simulink model "Quaternions_Method_main_davide"  (R2021b)
settings: Solver=ode4  StartTime=0.0  StopTime=Time  FixedStep=1e-2  RelTol=1e-13  AbsTol=1e-8
values from neighbouring files (symbols this model uses):
  a = 8.6251e+06    (= 8625100)    [Main.m]
  c = 299792*10^3    (= 299792000)    [Main.m]
  e = 0.1195    [Main.m]
  f_mag = 18    [Main.m]
  G = 6.67259 * 1e-11    (= 6.67259e-11)    [Main.m]
  H_0 = sqrt((g_1_0)^2 + (g_1_1)^2 + (h_1_1)^2)    [Main.m]
  i = 0.3815    [Main.m]
  MB = [2000; 0.3; 1; 0.12].*1e-2    [Main.m]
  muP = G*Mt    (= 398527110340000)    [Main.m]
  omega_0 = [om_x, om_y, om_z]    [Main.m]
  p_acc = 0.5    [Main.m]
  RD = 0.1*ones(1,10)    [Main.m]
  RS_MB = 0.5    [Main.m]
  RS_SP = 0.1    [Main.m]
  SP = [2000; 0.3; 1; 0.12].*1e-2    [Main.m]
  theta0 = 0    [Main.m]
  w_E = (2*pi)/(24*3600)    (= 7.27220521664e-05)    [Main.m]
undefined symbols (not defined in the file or in its folder): A_BN_0, A_rw, A_rw_star, H, magnitude, mr, rho_d_MB, rho_s_MB, sig_b, sig_n, T, t_sample
libraries: matrix_library x18, vrlib x8, simulink x2, simulink_extras x1
(part 3 of 6)

== system Quaternions_Method_main_davide/Sensors/Magnetometer1/Magnetometer  ==
  note: Questo blocco serve a verificare ortonrmalizzazione. Per verificare la amtrice in display deve avere daigonale 1
  A_BN : Inport
  Error Matrices : Subsystem
  Matrix Multiply : Product  Inputs=4  Multiplication=Matrix(*)
  RC Low Pass FIlter : Subsystem
  orthonormalization step 1 : Subsystem
  orthonormalization step 2 : Subsystem
  orthonormalization step 3 : Subsystem
  A_BN*_filtered : Outport
  A_BN*_not_filtered : Outport  Port=2
  wires:
  A_BN/1 -> Matrix Multiply/1
  Matrix Multiply/1 -> A_BN*_not_filtered/1, RC Low Pass FIlter/1(A*)
  Error Matrices/1(A_no) -> Matrix Multiply/2
  Error Matrices/2(A_sf) -> Matrix Multiply/3
  Error Matrices/3(A_noise) -> Matrix Multiply/4
  orthonormalization step 1/1(A_BN*_filtered) -> orthonormalization step 2/1(A*(t))
  RC Low Pass FIlter/1(A*_filtered) -> orthonormalization step 1/1(A*(t))
  orthonormalization step 2/1(A_BN*_filtered) -> orthonormalization step 3/1(A*(t))
  orthonormalization step 3/1(A_BN*_filtered) -> A_BN*_filtered/1

== system Quaternions_Method_main_davide/Sensors/Magnetometer1/b_B computation ==
  A_BN* : Inport
  b_N : Inport  Port=2
  Matrix Multiply : Product  Multiplication=Matrix(*)
  Saturation : Subsystem
  b_B : Outport
  wires:
  A_BN*/1 -> Matrix Multiply/1
  b_N/1 -> Matrix Multiply/2
  Matrix Multiply/1 -> Saturation/1(b_B)
  Saturation/1(b_B saturated) -> b_B/1

== system Quaternions_Method_main_davide/Sensors/Magnetometer1/model to reality difference ==
  A_BN : Inport
  A_BN* : Inport  Port=2
  b_N : Inport  Port=3
  A_BN*1 : Inport  Port=4
  A_BN1 : InportShadow
  MatrixMultiply{,1..3} (4 alike) : Product  Multiplication=Matrix(*)
  Scope : Scope  NumInputPorts=2
  Sum : Sum  Inputs=|-|+|
  Sum1 : Sum  Inputs=|-|+|
  b_N1 : InportShadow  Port=3
  wires:
  A_BN*/1 -> MatrixMultiply/1
  b_N/1 -> MatrixMultiply1/2, MatrixMultiply/2
  A_BN/1 -> MatrixMultiply1/1
  MatrixMultiply1/1 -> Sum/1
  MatrixMultiply/1 -> Sum/2
  Sum/1 -> Scope/1
  Sum1/1 -> Scope/2
  A_BN1/1 -> MatrixMultiply3/1
  MatrixMultiply3/1 -> Sum1/1
  A_BN*1/1 -> MatrixMultiply2/1
  MatrixMultiply2/1 -> Sum1/2
  b_N1/1 -> MatrixMultiply3/2, MatrixMultiply2/2

== system Quaternions_Method_main_davide/Sun Pointing 1/Pointing error with DCM/Desired attitude ==
  S_N : Inport
  Constant : Constant  Value=0
  Constant1 : Constant  Value=0
  Constant2 : Constant
  Cross Product : matrix_library/Cross Product
      settings: SourceProductBaseCode=SL
  Mux : Mux  Inputs=3
  Reshape : Reshape  OutputDimensionality=Column vector (2-D)
  Reshape1 : Reshape  OutputDimensionality=Customize  OutputDimensions=[3,3]
  Transpose : Math  Operator=transpose  SaturateOnIntegerOverflow=on
  Vector Concatenate : Concatenate  NumInputs=3
  Desired A_B_N : Outport
  wires:
  Constant/1 -> Mux/1
  Constant1/1 -> Mux/2
  Constant2/1 -> Mux/3
  Mux/1 -> Reshape/1
  Reshape/1 -> Vector Concatenate/3, Cross Product/1
  S_N/1 -> Cross Product/2, Vector Concatenate/2
  Cross Product/1 -> Vector Concatenate/1
  Vector Concatenate/1 -> Reshape1/1
  Reshape1/1 -> Transpose/1
  Transpose/1 -> Desired A_B_N/1

== system Quaternions_Method_main_davide/Sun Pointing 1/Pointing error with DCM/Detected pointing error ==
  Desired A_B_N : Inport
  A_B_N from attitude determination : Inport  Port=2
  Add : Sum  Inputs=+|+|+
  Add1 : Sum  Inputs=+|+|+
  Demux : Demux  Outputs=9
  Demux1 : Demux  Outputs=9
  Divide : Product  Inputs=*/
  Dot Product : DotProduct  InputSameDT=on  OutDataTypeStr=Inherit: Inherit via internal rule
  Gain : Gain  Gain=180/pi
  Mux : Mux  Inputs=3
  Mux1 : Mux  Inputs=3
  Power{,1..5} (6 alike) : Math  Operator=magnitude^2  SaturateOnIntegerOverflow=on
  Product : Product
  Reshape{,1..3} (4 alike) : Reshape  OutputDimensionality=Column vector (2-D)
  Sqrt : Sqrt  SaturateOnIntegerOverflow=on
  Terminator{,1..11} (12 alike) : Terminator
  Trigonometric Function : Trigonometry  Operator=acos
  detected pointing error : Outport
  wires:
  Desired A_B_N/1 -> Reshape/1
  Reshape/1 -> Demux/1
  Demux/1 -> Terminator/1
  Demux/2 -> [A21]
  Demux/3 -> Terminator1/1
  Demux/4 -> Terminator2/1
  Demux/6 -> Terminator3/1
  Demux/7 -> Terminator4/1
  Demux/8 -> [A23]
  Demux/9 -> Terminator5/1
  Demux1/7 -> Terminator10/1
  Demux1/6 -> Terminator9/1
  Demux1/5 -> [B22]
  Demux1/3 -> Terminator7/1
  Demux1/1 -> Terminator6/1
  Demux1/8 -> [B23]
  Demux1/4 -> Terminator8/1
  Reshape1/1 -> Demux1/1
  Demux1/2 -> [B21]
  Demux1/9 -> Terminator11/1
  A_B_N from attitude determination/1 -> Reshape1/1
  [A21] -> Power/1, Mux/1
  [A22] -> Mux/2, Power1/1
  [A23] -> Mux/3, Power2/1
  Mux/1 -> Reshape2/1
  Mux1/1 -> Reshape3/1
  [B22] -> Mux1/2, Power4/1
  [B21] -> Power5/1, Mux1/1
  [B23] -> Mux1/3, Power3/1
  Reshape2/1 -> Dot Product/1
  Reshape3/1 -> Dot Product/2
  Dot Product/1 -> Divide/1
  Power1/1 -> Add/2
  Power2/1 -> Add/1
  Power/1 -> Add/3
  Add/1 -> Sqrt/1
  Sqrt/1 -> Product/1
  Power4/1 -> Add1/2
  Power5/1 -> Add1/1
  Power3/1 -> Add1/3
  Add1/1 -> Product/2
  Product/1 -> Divide/2
  Divide/1 -> Trigonometric Function/1
  Trigonometric Function/1 -> Gain/1
  Gain/1 -> detected pointing error/1
  Demux/5 -> [A22]

== system Quaternions_Method_main_davide/Sun Pointing 1/Pointing error with DCM/Real pointing error ==
  " A_B_N from Euler" : Inport
  Desired A_B_N : Inport  Port=2
  Add : Sum  Inputs=+|+|+
  Add1 : Sum  Inputs=+|+|+
  Demux : Demux  Outputs=9
  Demux1 : Demux  Outputs=9
  Divide : Product  Inputs=/*
  Dot Product : DotProduct  InputSameDT=on  OutDataTypeStr=Inherit: Inherit via internal rule
  Mux : Mux  Inputs=3
  Mux1 : Mux  Inputs=3
  Power{,1..5} (6 alike) : Math  Operator=magnitude^2  SaturateOnIntegerOverflow=on
  Product : Product
  Reshape{,1..3} (4 alike) : Reshape  OutputDimensionality=Column vector (2-D)
  Sqrt : Sqrt  SaturateOnIntegerOverflow=on
  Terminator{,1..11} (12 alike) : Terminator
  Trigonometric Function : Trigonometry  Operator=acos
  real pointing error : Outport
  wires:
  Divide/1 -> Trigonometric Function/1
  Product/1 -> Divide/1
  Add1/1 -> Product/2
  Power3/1 -> Add1/3
  Power5/1 -> Add1/1
  Power4/1 -> Add1/2
  Sqrt/1 -> Product/1
  Add/1 -> Sqrt/1
  Power/1 -> Add/3
  Power2/1 -> Add/1
  Power1/1 -> Add/2
  Dot Product/1 -> Divide/2
  Reshape3/1 -> Dot Product/2
  Reshape2/1 -> Dot Product/1
  [B23] -> Power3/1, Mux1/3
  [B21] -> Mux1/1, Power5/1
  [B22] -> Power4/1, Mux1/2
  Mux1/1 -> Reshape3/1
  Mux/1 -> Reshape2/1
  [A23] -> Power2/1, Mux/3
  [A22] -> Power1/1, Mux/2
  [A21] -> Mux/1, Power/1
  Desired A_B_N/1 -> Reshape1/1
  Demux1/9 -> Terminator11/1
  Demux1/2 -> [B21]
  Reshape1/1 -> Demux1/1
  Demux1/4 -> Terminator8/1
  Demux1/8 -> [B23]
  Demux1/1 -> Terminator6/1
  Demux1/3 -> Terminator7/1
  Demux1/5 -> [B22]
  Demux1/6 -> Terminator9/1
  Demux1/7 -> Terminator10/1
  Demux/9 -> Terminator5/1
  Demux/8 -> [A23]
  Demux/7 -> Terminator4/1
  Demux/6 -> Terminator3/1
  Demux/5 -> [A22]
  Demux/4 -> Terminator2/1
  Demux/3 -> Terminator1/1
  Demux/2 -> [A21]
  Demux/1 -> Terminator/1
  Reshape/1 -> Demux/1
  " A_B_N from Euler"/1 -> Reshape/1
  Trigonometric Function/1 -> real pointing error/1

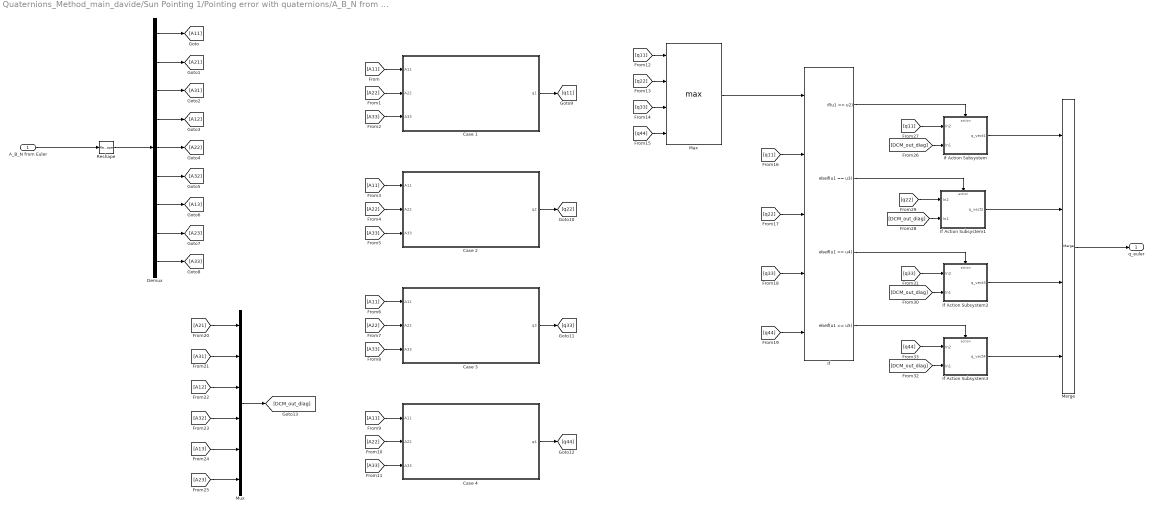
== system Quaternions_Method_main_davide/Sun Pointing 1/Pointing error with quaternions/A_B_N from Euler to quaternion ==
  A_B_N from Euler : Inport
  Case 1 : Subsystem
  Case 2 : Subsystem
  Case 3 : Subsystem
  Case 4 : Subsystem
  Demux : Demux  Outputs=9
  If : If  NumInputs=5  IfExpression=u1 == u2  ElseIfExpressions=u1 == u3, u1 == u4, u1 == u5  ShowElse=off
  If Action Subsystem : Subsystem  TreatAsAtomicUnit=on
  If Action Subsystem1 : Subsystem  TreatAsAtomicUnit=on
  If Action Subsystem2 : Subsystem  TreatAsAtomicUnit=on
  If Action Subsystem3 : Subsystem  TreatAsAtomicUnit=on
  Max : MinMax  Function=max  Inputs=4
  Merge : Merge  Inputs=4
  Mux : Mux  Inputs=6
  Reshape : Reshape  OutputDimensionality=Column vector (2-D)
  q_euler : Outport
  wires:
  A_B_N from Euler/1 -> Reshape/1
  Reshape/1 -> Demux/1
  Demux/1 -> [A11]
  Demux/2 -> [A21]
  Demux/3 -> [A31]
  Demux/4 -> [A12]
  Demux/5 -> [A22]
  Demux/6 -> [A32]
  Demux/7 -> [A13]
  Demux/8 -> [A23]
  Demux/9 -> [A33]
  [A22] -> Case 1/2(A22)
  [A33] -> Case 1/3(A33)
  [A11] -> Case 1/1(A11)
  [A11] -> Case 2/1(A11)
  [A33] -> Case 2/3(A33)
  [A22] -> Case 2/2(A22)
  [A22] -> Case 3/2(A22)
  [A33] -> Case 3/3(A33)
  [A11] -> Case 3/1(A11)
  [A11] -> Case 4/1(A11)
  [A33] -> Case 4/3(A33)
  [A22] -> Case 4/2(A22)
  Case 1/1(q1) -> [q11]
  Case 2/1(q2) -> [q22]
  Case 3/1(q3) -> [q33]
  Case 4/1(q4) -> [q44]
  [q11] -> Max/1
  [q33] -> Max/3
  [q22] -> Max/2
  [q44] -> Max/4
  Max/1 -> If/1
  [q11] -> If/2
  [q22] -> If/3
  [q33] -> If/4
  [q44] -> If/5
  If/1 -> If Action Subsystem/Action
  If/2 -> If Action Subsystem1/Action
  If/3 -> If Action Subsystem2/Action
  If/4 -> If Action Subsystem3/Action
  If Action Subsystem3/1(q_vect4) -> Merge/4
  If Action Subsystem2/1(q_vect3) -> Merge/3
  If Action Subsystem1/1(q_vect2) -> Merge/2
  If Action Subsystem/1(q_vect1) -> Merge/1
  Merge/1 -> q_euler/1
  [A23] -> Mux/6
  [A13] -> Mux/5
  [A32] -> Mux/4
  [A12] -> Mux/3
  [A31] -> Mux/2
  [A21] -> Mux/1
  Mux/1 -> [DCM_out_diag]
  [DCM_out_diag] -> If Action Subsystem/2(In1)
  [q11] -> If Action Subsystem/1(In2)
  [q22] -> If Action Subsystem1/1(In2)
  [DCM_out_diag] -> If Action Subsystem1/2(In1)
  [DCM_out_diag] -> If Action Subsystem2/2(In1)
  [q33] -> If Action Subsystem2/1(In2)
  [q44] -> If Action Subsystem3/1(In2)
  [DCM_out_diag] -> If Action Subsystem3/2(In1)

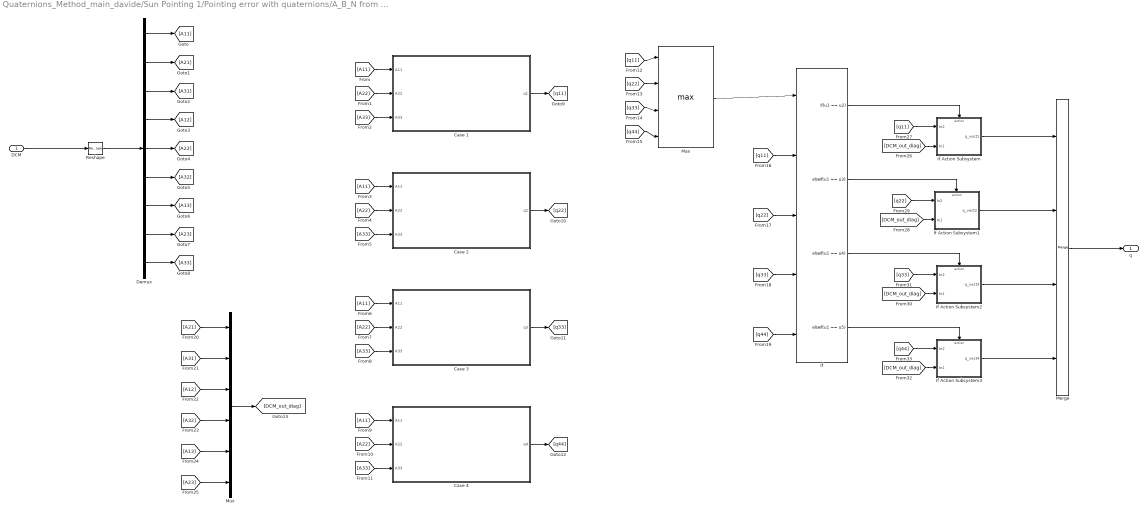
== system Quaternions_Method_main_davide/Sun Pointing 1/Pointing error with quaternions/A_B_N from attitude det to quaternion2 ==
  DCM : Inport
  Case 1 : Subsystem
  Case 2 : Subsystem
  Case 3 : Subsystem
  Case 4 : Subsystem
  Demux : Demux  Outputs=9
  If : If  NumInputs=5  IfExpression=u1 == u2  ElseIfExpressions=u1 == u3, u1 == u4, u1 == u5  ShowElse=off
  If Action Subsystem : Subsystem  TreatAsAtomicUnit=on
  If Action Subsystem1 : Subsystem  TreatAsAtomicUnit=on
  If Action Subsystem2 : Subsystem  TreatAsAtomicUnit=on
  If Action Subsystem3 : Subsystem  TreatAsAtomicUnit=on
  Max : MinMax  Function=max  Inputs=4
  Merge : Merge  Inputs=4
  Mux : Mux  Inputs=6
  Reshape : Reshape  OutputDimensionality=Column vector (2-D)
  q : Outport
  wires:
  [DCM_out_diag] -> If Action Subsystem3/2(In1)
  [q44] -> If Action Subsystem3/1(In2)
  [q33] -> If Action Subsystem2/1(In2)
  [DCM_out_diag] -> If Action Subsystem2/2(In1)
  [DCM_out_diag] -> If Action Subsystem1/2(In1)
  [q22] -> If Action Subsystem1/1(In2)
  [q11] -> If Action Subsystem/1(In2)
  [DCM_out_diag] -> If Action Subsystem/2(In1)
  Mux/1 -> [DCM_out_diag]
  [A21] -> Mux/1
  [A31] -> Mux/2
  [A12] -> Mux/3
  [A32] -> Mux/4
  [A13] -> Mux/5
  [A23] -> Mux/6
  Merge/1 -> q/1
  If Action Subsystem/1(q_vect1) -> Merge/1
  If Action Subsystem1/1(q_vect2) -> Merge/2
  If Action Subsystem2/1(q_vect3) -> Merge/3
  If Action Subsystem3/1(q_vect4) -> Merge/4
  If/4 -> If Action Subsystem3/Action
  If/3 -> If Action Subsystem2/Action
  If/2 -> If Action Subsystem1/Action
  If/1 -> If Action Subsystem/Action
  [q44] -> If/5
  [q33] -> If/4
  [q22] -> If/3
  [q11] -> If/2
  Max/1 -> If/1
  [q44] -> Max/4
  [q22] -> Max/2
  [q33] -> Max/3
  [q11] -> Max/1
  Case 4/1(q4) -> [q44]
  Case 3/1(q3) -> [q33]
  Case 2/1(q2) -> [q22]
  Case 1/1(q1) -> [q11]
  [A22] -> Case 4/2(A22)
  [A33] -> Case 4/3(A33)
  [A11] -> Case 4/1(A11)
  [A11] -> Case 3/1(A11)
  [A33] -> Case 3/3(A33)
  [A22] -> Case 3/2(A22)
  [A22] -> Case 2/2(A22)
  [A33] -> Case 2/3(A33)
  [A11] -> Case 2/1(A11)
  [A11] -> Case 1/1(A11)
  [A33] -> Case 1/3(A33)
  [A22] -> Case 1/2(A22)
  Demux/9 -> [A33]
  Demux/8 -> [A23]
  Demux/7 -> [A13]
  Demux/6 -> [A32]
  Demux/5 -> [A22]
  Demux/4 -> [A12]
  Demux/3 -> [A31]
  Demux/2 -> [A21]
  Demux/1 -> [A11]
  Reshape/1 -> Demux/1
  DCM/1 -> Reshape/1

== system Quaternions_Method_main_davide/Sun Pointing 1/Pointing error with quaternions/Desired attitude ==
  S_N : Inport
  Constant : Constant  Value=0
  Constant1 : Constant  Value=0
  Constant2 : Constant
  Cross Product : matrix_library/Cross Product
      settings: SourceProductBaseCode=SL
  Mux : Mux  Inputs=3
  Reshape : Reshape  OutputDimensionality=Column vector (2-D)
  Reshape1 : Reshape  OutputDimensionality=Customize  OutputDimensions=[3,3]
  Transpose : Math  Operator=transpose  SaturateOnIntegerOverflow=on
  Vector Concatenate : Concatenate  NumInputs=3
  Desired A_B_N : Outport
  wires:
  Constant/1 -> Mux/1
  Constant1/1 -> Mux/2
  Constant2/1 -> Mux/3
  Mux/1 -> Reshape/1
  Reshape/1 -> Cross Product/2, Vector Concatenate/3
  S_N/1 -> Vector Concatenate/2, Cross Product/1
  Cross Product/1 -> Vector Concatenate/1
  Vector Concatenate/1 -> Reshape1/1
  Reshape1/1 -> Transpose/1
  Transpose/1 -> Desired A_B_N/1

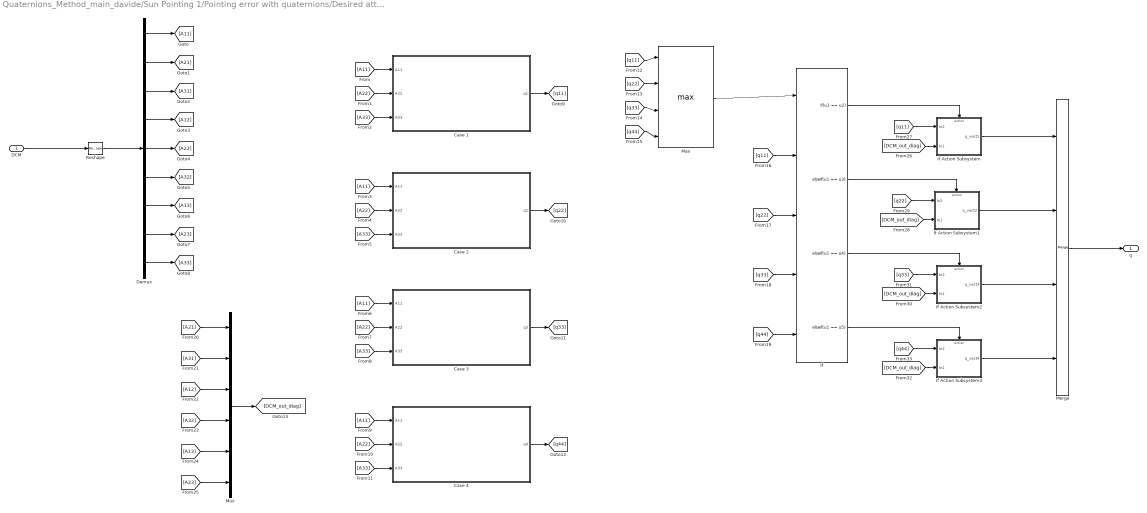
== system Quaternions_Method_main_davide/Sun Pointing 1/Pointing error with quaternions/Desired attitude to quaternion1 ==
  DCM : Inport
  Case 1 : Subsystem
  Case 2 : Subsystem
  Case 3 : Subsystem
  Case 4 : Subsystem
  Demux : Demux  Outputs=9
  If : If  NumInputs=5  IfExpression=u1 == u2  ElseIfExpressions=u1 == u3, u1 == u4, u1 == u5  ShowElse=off
  If Action Subsystem : Subsystem  TreatAsAtomicUnit=on
  If Action Subsystem1 : Subsystem  TreatAsAtomicUnit=on
  If Action Subsystem2 : Subsystem  TreatAsAtomicUnit=on
  If Action Subsystem3 : Subsystem  TreatAsAtomicUnit=on
  Max : MinMax  Function=max  Inputs=4
  Merge : Merge  Inputs=4
  Mux : Mux  Inputs=6
  Reshape : Reshape  OutputDimensionality=Column vector (2-D)
  q : Outport
  wires:
  DCM/1 -> Reshape/1
  Reshape/1 -> Demux/1
  Demux/1 -> [A11]
  Demux/2 -> [A21]
  Demux/3 -> [A31]
  Demux/4 -> [A12]
  Demux/5 -> [A22]
  Demux/6 -> [A32]
  Demux/7 -> [A13]
  Demux/8 -> [A23]
  Demux/9 -> [A33]
  [A22] -> Case 1/2(A22)
  [A33] -> Case 1/3(A33)
  [A11] -> Case 1/1(A11)
  [A11] -> Case 2/1(A11)
  [A33] -> Case 2/3(A33)
  [A22] -> Case 2/2(A22)
  [A22] -> Case 3/2(A22)
  [A33] -> Case 3/3(A33)
  [A11] -> Case 3/1(A11)
  [A11] -> Case 4/1(A11)
  [A33] -> Case 4/3(A33)
  [A22] -> Case 4/2(A22)
  Case 1/1(q1) -> [q11]
  Case 2/1(q2) -> [q22]
  Case 3/1(q3) -> [q33]
  Case 4/1(q4) -> [q44]
  [q11] -> Max/1
  [q33] -> Max/3
  [q22] -> Max/2
  [q44] -> Max/4
  Max/1 -> If/1
  [q11] -> If/2
  [q22] -> If/3
  [q33] -> If/4
  [q44] -> If/5
  If/1 -> If Action Subsystem/Action
  If/2 -> If Action Subsystem1/Action
  If/3 -> If Action Subsystem2/Action
  If/4 -> If Action Subsystem3/Action
  If Action Subsystem3/1(q_vect4) -> Merge/4
  If Action Subsystem2/1(q_vect3) -> Merge/3
  If Action Subsystem1/1(q_vect2) -> Merge/2
  If Action Subsystem/1(q_vect1) -> Merge/1
  Merge/1 -> q/1
  [A23] -> Mux/6
  [A13] -> Mux/5
  [A32] -> Mux/4
  [A12] -> Mux/3
  [A31] -> Mux/2
  [A21] -> Mux/1
  Mux/1 -> [DCM_out_diag]
  [DCM_out_diag] -> If Action Subsystem/2(In1)
  [q11] -> If Action Subsystem/1(In2)
  [q22] -> If Action Subsystem1/1(In2)
  [DCM_out_diag] -> If Action Subsystem1/2(In1)
  [DCM_out_diag] -> If Action Subsystem2/2(In1)
  [q33] -> If Action Subsystem2/1(In2)
  [q44] -> If Action Subsystem3/1(In2)
  [DCM_out_diag] -> If Action Subsystem3/2(In1)

== system Quaternions_Method_main_davide/Enviroment/Magnetic torque /Magnetic field in body frame/Direction of M field ==
  Clock : Clock
  Constant : Constant  Value=eps
  Constant1 : Constant  Value=w_E
  Mux : Mux  Inputs=3
  Product : Product
  Product1 : Product
  Product2 : Product
  Reshape : Reshape  OutputDimensionality=Column vector (2-D)
  Trigonometric Function : Trigonometry
  Trigonometric Function1 : Trigonometry  Operator=cos
  Trigonometric Function2 : Trigonometry  Operator=cos
  Trigonometric Function3 : Trigonometry
  m_vect : Outport
  wires:
  Constant1/1 -> Product/1
  Clock/1 -> Product/2
  Constant/1 -> Trigonometric Function2/1, Trigonometric Function/1
  Product/1 -> Trigonometric Function3/1, Trigonometric Function1/1
  Trigonometric Function/1 -> Product2/1, Product1/1
  Trigonometric Function1/1 -> Product1/2
  Trigonometric Function3/1 -> Product2/2
  Product1/1 -> Mux/1
  Product2/1 -> Mux/2
  Trigonometric Function2/1 -> Mux/3
  Mux/1 -> Reshape/1
  Reshape/1 -> m_vect/1

== system Quaternions_Method_main_davide/Enviroment/Solar Radiation Perturbation/Force/MB Forces ==
  P : Inport
  S_B : Inport  Port=2
  RD_MB : Inport  Port=3
  N_MB : Inport  Port=4
  M_B : Inport  Port=5
  Add : Sum
  Constant : Constant
  Constant10 : Constant  Value=[1,1,1,1,1,1]
  Constant14 : Constant  Value=[1 1 1]
  Constant4 : Constant  Value=RS_MB
  Constant8 : Constant  Value=[1 1 1]
  Constant9 : Constant  Value=[1 1 1]
  Dot Product N*MB : Subsystem
  Gain : Gain  Gain=-1
  Gain1 : Gain  Gain=2
  Gain2 : Gain  Gain=2/3
  Matrix Multiply{,1,4,6} (4 alike) : Product  Multiplication=Matrix(*)
  Product : Product  Inputs=4
  Product1 : Product
  Product2 : Product
  Product3 : Product
  Reshape : Reshape  OutputDimensionality=Column vector (2-D)
  Reshape1 : Reshape  OutputDimensionality=Row vector (2-D)
  Reshape14 : Reshape  OutputDimensionality=Column vector (2-D)
  Reshape2 : Reshape  OutputDimensionality=Row vector (2-D)
  Reshape7 : Reshape  OutputDimensionality=Row vector (2-D)
  Sum : Sum  Inputs=+-
  Sum1 : Sum
  Vector Concatenate6 : Concatenate  NumInputs=6
  creation of the areas of the S/C : Subsystem
  F_MB : Outport
  A_MB : Outport  Port=2
  prodsca_MB : Outport  Port=3
  wires:
  Constant4/1 -> Sum/2, Gain1/1
  Matrix Multiply6/1 -> Add/1
  Vector Concatenate6/1 -> Reshape14/1
  Constant9/1 -> Reshape1/1
  Reshape1/1 -> Matrix Multiply1/2
  Constant/1 -> Sum/1
  Reshape2/1 -> Matrix Multiply/2
  Gain/1 -> Product/1
  [S_B] -> Product1/1
  Sum/1 -> Product1/2
  creation of the areas of the S/C/1(a*b_1) -> Vector Concatenate6/1
  Add/1 -> Product/4
  Constant8/1 -> Reshape2/1
  Gain2/1 -> Sum1/2
  [dot_N_MB_SB] -> prodsca_MB/1
  [RD_MB] -> Gain2/1
  creation of the areas of the S/C/2(a*b_2) -> Vector Concatenate6/2
  [P] -> Gain/1
  Product2/1 -> Sum1/1
  Matrix Multiply/1 -> Product3/2
  [dot_N_MB_SB] -> Matrix Multiply1/1
  Matrix Multiply4/1 -> Product/2
  Reshape14/1 -> A_MB/1, Matrix Multiply4/1
  Matrix Multiply1/1 -> Product/3
  Gain1/1 -> Product2/2
  Sum1/1 -> Matrix Multiply/1
  creation of the areas of the S/C/4(a*h_2) -> Vector Concatenate6/4
  [dot_N_MB_SB] -> Product2/1
  creation of the areas of the S/C/5(b*h_1) -> Vector Concatenate6/5
  creation of the areas of the S/C/6(b*h_2) -> Vector Concatenate6/6
  Product1/1 -> Matrix Multiply6/2
  creation of the areas of the S/C/3(a*h_1) -> Vector Concatenate6/3
  [MB] -> creation of the areas of the S/C/1(MB)
  Constant14/1 -> Reshape7/1
  Product/1 -> F_MB/1
  Reshape7/1 -> Matrix Multiply4/2
  Product3/1 -> Add/2
  Constant10/1 -> Reshape/1
  Reshape/1 -> Matrix Multiply6/1
  [N_MB] -> Product3/1
  Dot Product N*MB/1(Out1) -> [dot_N_MB_SB]
  S_B/1 -> [S_B]
  RD_MB/1 -> [RD_MB]
  P/1 -> [P]
  N_MB/1 -> [N_MB]
  M_B/1 -> [MB]
  [S_B] -> Dot Product N*MB/1(S_B)
  [N_MB] -> Dot Product N*MB/2(N_MB)

== system Quaternions_Method_main_davide/Enviroment/Solar Radiation Perturbation/Force/SP Forces ==
  P : Inport
  S_B : Inport  Port=2
  RD_SP : Inport  Port=3
  N_SP : Inport  Port=4
  SP : Inport  Port=5
  Add1 : Sum
  Constant1 : Constant
  Constant12 : Constant  Value=[1 1 1]
  Constant13 : Constant  Value=[1 1 1]
  Constant14 : Constant  Value=[1 1 1]
  Constant15 : Constant  Value=[1,1,1,1]
  Constant5 : Constant  Value=RS_SP
  Dot Product N*SP : Subsystem
  Gain4 : Gain  Gain=-1
  Gain5 : Gain  Gain=2
  Gain6 : Gain  Gain=2/3
  Matrix Multiply{2..4,8} (4 alike) : Product  Multiplication=Matrix(*)
  Product4 : Product  Inputs=4
  Product5 : Product
  Product6 : Product
  Product7 : Product
  Reshape14 : Reshape  OutputDimensionality=Column vector (2-D)
  Reshape3 : Reshape  OutputDimensionality=Row vector (2-D)
  Reshape6 : Reshape  OutputDimensionality=Row vector (2-D)
  Reshape7 : Reshape  OutputDimensionality=Row vector (2-D)
  Reshape9 : Reshape  OutputDimensionality=Column vector (2-D)
  Sum3 : Sum  Inputs=+-
  Sum4 : Sum
  Vector Concatenate6 : Concatenate  NumInputs=4
  creation of the areas of the S/C : Subsystem
  F_SP : Outport
  prodscal_SP1 : Outport  Port=2
  wires:
  Sum3/1 -> Product5/2
  Reshape3/1 -> Matrix Multiply2/2
  Constant13/1 -> Reshape6/1
  Gain4/1 -> Product4/1
  Product6/1 -> Sum4/1
  Constant12/1 -> Reshape3/1
  [S_B] -> Product5/1
  [P] -> Gain4/1
  Gain6/1 -> Sum4/2
  [RD_SP] -> Gain6/1
  [N_SP] -> Product7/1
  Constant1/1 -> Sum3/1
  Constant15/1 -> Reshape9/1
  Sum4/1 -> Matrix Multiply3/1
  Product4/1 -> F_SP/1
  Constant5/1 -> Gain5/1, Sum3/2
  [dot_N_SP_SB] -> Matrix Multiply2/1
  Reshape6/1 -> Matrix Multiply3/2
  Product5/1 -> Matrix Multiply8/2
  Matrix Multiply3/1 -> Product7/2
  Gain5/1 -> Product6/2
  Matrix Multiply2/1 -> Product4/3
  Reshape9/1 -> Matrix Multiply8/1
  Product7/1 -> Add1/2
  [dot_N_SP_SB] -> Product6/1
  Add1/1 -> Product4/4
  [dot_N_SP_SB] -> prodscal_SP1/1
  Matrix Multiply8/1 -> Add1/1
  S_B/1 -> [S_B]
  N_SP/1 -> [N_SP]
  P/1 -> [P]
  SP/1 -> [SP]
  RD_SP/1 -> [RD_SP]
  Matrix Multiply4/1 -> Product4/2
  Vector Concatenate6/1 -> Reshape14/1
  Reshape14/1 -> Matrix Multiply4/1
  Constant14/1 -> Reshape7/1
  [SP] -> creation of the areas of the S/C/1(SP)
  Reshape7/1 -> Matrix Multiply4/2
  creation of the areas of the S/C/1(a*b_1) -> Vector Concatenate6/1
  creation of the areas of the S/C/2(a*b_2) -> Vector Concatenate6/2
  creation of the areas of the S/C/3(a*b_3) -> Vector Concatenate6/3
  creation of the areas of the S/C/4(a*b_4) -> Vector Concatenate6/4
  [S_B] -> Dot Product N*SP/1(S_B)
  [N_SP] -> Dot Product N*SP/2(N_SP)
  Dot Product N*SP/1(dot_N_SP_SB) -> [dot_N_SP_SB]

== system Quaternions_Method_main_davide/Enviroment/Solar Radiation Perturbation/Force MB/Subsystem ==
  S_B : Inport
  N_MB : Inport  Port=2
  Constant3 : Constant  Value=[1, 1, 1]
  Matrix Multiply5 : Product  Multiplication=Matrix(*)
  Product10 : Product
  Reshape11 : Reshape  OutputDimensionality=Row vector (2-D)
  Reshape12 : Reshape  OutputDimensionality=Column vector (2-D)
  Sum of Elements : Sum  Inputs=+  CollapseMode=Specified dimension  CollapseDim=2
  Out1 : Outport
  wires:
  Matrix Multiply5/1 -> Product10/1
  Reshape12/1 -> Matrix Multiply5/1
  S_B/1 -> Reshape12/1
  Product10/1 -> Sum of Elements/1
  N_MB/1 -> Product10/2
  Sum of Elements/1 -> Out1/1
  Constant3/1 -> Reshape11/1
  Reshape11/1 -> Matrix Multiply5/2

== system Quaternions_Method_main_davide/Enviroment/Solar Radiation Perturbation/S_B dot N_MB/If Action Subsystem ==
  NMB : Inport
  Action Port : ActionPort
  Constant : Constant
  Selector : Selector  NumberOfDimensions=2  InputPortWidth=3  IndexOptions=Index vector (dialog),Index vector (dialog)  Indices=1,[1 2 3]  OutputSizes=1,1
  x : Outport
  pointer : Outport  Port=2
  wires:
  NMB/1 -> Selector/1
  Selector/1 -> x/1
  Constant/1 -> pointer/1

== system Quaternions_Method_main_davide/Enviroment/Solar Radiation Perturbation/S_B dot N_MB/If Action Subsystem1 ==
  NMB : Inport
  Action Port : ActionPort
  Constant : Constant
  Selector : Selector  NumberOfDimensions=2  InputPortWidth=3  IndexOptions=Index vector (dialog),Index vector (dialog)  Indices=2,[1 2 3]  OutputSizes=1,1
  y : Outport
  pointer : Outport  Port=2
  wires:
  Selector/1 -> y/1
  NMB/1 -> Selector/1
  Constant/1 -> pointer/1

== system Quaternions_Method_main_davide/Enviroment/Solar Radiation Perturbation/S_B dot N_MB/If Action Subsystem2 ==
  NMB : Inport
  Action Port : ActionPort
  Constant : Constant
  Selector : Selector  NumberOfDimensions=2  InputPortWidth=3  IndexOptions=Index vector (dialog),Index vector (dialog)  Indices=3,[1 2 3]  OutputSizes=1,1
  z : Outport
  pointer : Outport  Port=2
  wires:
  NMB/1 -> Selector/1
  Selector/1 -> z/1
  Constant/1 -> pointer/1

== system Quaternions_Method_main_davide/Enviroment/Solar Radiation Perturbation/S_B dot N_MB/If Action Subsystem3 ==
  NMB : Inport
  Action Port : ActionPort
  Constant : Constant  Value=-1
  Selector : Selector  NumberOfDimensions=2  InputPortWidth=3  IndexOptions=Index vector (dialog),Index vector (dialog)  Indices=4,[1 2 3]  OutputSizes=1,1
  -x : Outport
  pointer : Outport  Port=2
  wires:
  Selector/1 -> -x/1
  NMB/1 -> Selector/1
  Constant/1 -> pointer/1

== system Quaternions_Method_main_davide/Enviroment/Solar Radiation Perturbation/S_B dot N_MB/If Action Subsystem4 ==
  NMB : Inport
  Action Port : ActionPort
  Constant : Constant  Value=-1
  Selector : Selector  NumberOfDimensions=2  InputPortWidth=3  IndexOptions=Index vector (dialog),Index vector (dialog)  Indices=5,[1 2 3]  OutputSizes=1,1
  -y : Outport
  pointer : Outport  Port=2
  wires:
  NMB/1 -> Selector/1
  Selector/1 -> -y/1
  Constant/1 -> pointer/1

== system Quaternions_Method_main_davide/Enviroment/Solar Radiation Perturbation/S_B dot N_MB/If Action Subsystem5 ==
  NMB : Inport
  Action Port : ActionPort
  Constant : Constant  Value=-1
  Selector : Selector  NumberOfDimensions=2  InputPortWidth=3  IndexOptions=Index vector (dialog),Index vector (dialog)  Indices=6,[1 2 3]  OutputSizes=1,1
  -z : Outport
  pointer : Outport  Port=2
  wires:
  Selector/1 -> -z/1
  NMB/1 -> Selector/1
  Constant/1 -> pointer/1

== system Quaternions_Method_main_davide/Enviroment/Solar Radiation Perturbation/Sum forces/determine highlighted area ==
  note: matrice che ha per colonne i vettori distanza tra il CM del MB e i centri geom delle aree illuminate dal sole
  MB : Inport
  A_MB : Inport  Port=2
  prodscal_MB(tra norm e sun direction) : Inport  Port=3
  S_B : Inport  Port=4
  Demux1 : Demux  Outputs=6
  Demux2 : Demux  Outputs=6
  If : If  NumInputs=2  IfExpression=u1>0  ElseIfExpressions=u2>0
  If Action Subsystem : Subsystem  TreatAsAtomicUnit=on
  If Action Subsystem1 : Subsystem  TreatAsAtomicUnit=on
  If Action Subsystem2 : Subsystem  TreatAsAtomicUnit=on
  If Action Subsystem3 : Subsystem  TreatAsAtomicUnit=on
  If Action Subsystem4 : Subsystem  TreatAsAtomicUnit=on
  If Action Subsystem5 : Subsystem  TreatAsAtomicUnit=on
  If Action Subsystem6 : Subsystem  TreatAsAtomicUnit=on
  If Action Subsystem7 : Subsystem  TreatAsAtomicUnit=on
  If Action Subsystem8 : Subsystem  TreatAsAtomicUnit=on
  If1 : If  NumInputs=2  IfExpression=u1>0  ElseIfExpressions=u2>0
  If2 : If  NumInputs=2  IfExpression=u1>0  ElseIfExpressions=u2>0
  Merge : Merge  Inputs=3
  Merge1 : Merge  Inputs=3
  Merge2 : Merge  Inputs=3
  Mux : Mux  Inputs=3
  Product{10..15} (6 alike) : Product
  Reshape : Reshape  OutputDimensionality=Column vector (2-D)
  Reshape1 : Reshape  OutputDimensionality=Column vector (2-D)
  "creazione della matrice che ha per colonne i vettori distanza tra il CM del MB e i centri geom delle aree illuminate dal sole " : Subsystem
  distance matrix : Outport
  wires:
  Reshape/1 -> Demux2/1
  prodscal_MB(tra norm e sun direction)/1 -> Reshape/1
  Demux2/1 -> Product15/2  "x"
  Demux2/2 -> Product13/2  "y"
  Demux2/3 -> Product12/2  "z"
  Demux2/4 -> Product11/2  "-x"
  Demux2/5 -> Product10/2  "-y"
  Demux2/6 -> Product14/2  "-z"
  Demux1/1 -> Product12/1
  Mux/1 -> Reshape1/1
  Product15/1 -> If Action Subsystem/1(In1), If/1  "x"
  If/1 -> If Action Subsystem/Action
  Reshape1/1 -> "creazione della matrice che ha per colonne i vettori distanza tra il CM del MB e i centri geom delle aree illuminate dal sole "/2(A_vect)  "Areas_vect = vettore contenente le aree nelle direzioni x, y, z, -x, -y, -z"
  "creazione della matrice che ha per colonne i vettori distanza tra il CM del MB e i centri geom delle aree illuminate dal sole "/1(distance matrix) -> distance matrix/1
  A_MB/1 -> Demux1/1
  Demux1/2 -> Product14/1
  Demux1/3 -> Product13/1
  Demux1/4 -> Product10/1
  Demux1/5 -> Product15/1
  Demux1/6 -> Product11/1
  If/2 -> If Action Subsystem1/Action
  Product11/1 -> If Action Subsystem1/1(In1), If/2  "-x"
  If1/2 -> If Action Subsystem4/Action
  If1/3 -> If Action Subsystem5/Action
  If1/1 -> If Action Subsystem3/Action
  Product10/1 -> If Action Subsystem4/1(In1), If1/2  "-y"
  Product13/1 -> If Action Subsystem3/1(In1), If1/1  "y"
  If2/2 -> If Action Subsystem7/Action
  If2/3 -> If Action Subsystem8/Action
  If2/1 -> If Action Subsystem6/Action
  Product12/1 -> If Action Subsystem6/1(In1), If2/1  "z"
  Product14/1 -> If Action Subsystem7/1(In1), If2/2  "-z"
  Merge/1 -> Mux/2
  Merge2/1 -> Mux/3
  Merge1/1 -> Mux/1
  If Action Subsystem8/1(Out1) -> Merge2/3
  If Action Subsystem7/1(Out1) -> Merge2/2
  If Action Subsystem6/1(Out1) -> Merge2/1
  If Action Subsystem5/1(Out1) -> Merge/3
  If Action Subsystem4/1(Out1) -> Merge/2
  MB/1 -> "creazione della matrice che ha per colonne i vettori distanza tra il CM del MB e i centri geom delle aree illuminate dal sole "/1(MB)
  If Action Subsystem/1(Out1) -> Merge1/1
  If Action Subsystem1/1(Out1) -> Merge1/2
  If/3 -> If Action Subsystem2/Action
  If Action Subsystem2/1(Out1) -> Merge1/3
  If Action Subsystem3/1(Out1) -> Merge/1
  S_B/1 -> [S_B]
  [S_B] -> "creazione della matrice che ha per colonne i vettori distanza tra il CM del MB e i centri geom delle aree illuminate dal sole "/3(S_B)

== system Quaternions_Method_main_davide/Enviroment/Solar Radiation Perturbation/Sum forces/determine highlighted area1 ==
  prodscal_SP(tra norm e sun direction) : Inport
  Demux2 : Demux
  If : If  NumInputs=2  IfExpression=u1>0  ElseIfExpressions=u2>0
  If Action Subsystem : Subsystem  TreatAsAtomicUnit=on
  If Action Subsystem1 : Subsystem  TreatAsAtomicUnit=on
  If Action Subsystem2 : Subsystem  TreatAsAtomicUnit=on
  If Action Subsystem3 : Subsystem  TreatAsAtomicUnit=on
  If Action Subsystem4 : Subsystem  TreatAsAtomicUnit=on
  If Action Subsystem5 : Subsystem  TreatAsAtomicUnit=on
  If1 : If  NumInputs=2  IfExpression=u1>0  ElseIfExpressions=u2>0
  Merge : Merge  Inputs=3
  Merge1 : Merge  Inputs=3
  Mux : Mux  Inputs=2
  Reshape : Reshape  OutputDimensionality=Column vector (2-D)
  Reshape1 : Reshape  OutputDimensionality=Column vector (2-D)
  face illuminated : Outport
  wires:
  If Action Subsystem2/1(Out1) -> Merge/3
  If/3 -> If Action Subsystem2/Action
  Merge/1 -> Mux/1
  Demux2/1 -> If/1  "y_1"
  Mux/1 -> Reshape1/1
  Demux2/2 -> If/2  "-y_1"
  prodscal_SP(tra norm e sun direction)/1 -> Reshape/1
  Reshape/1 -> Demux2/1
  Demux2/3 -> If1/1  "y_2"
  Demux2/4 -> If1/2  "-y_2"
  Merge1/1 -> Mux/2
  Reshape1/1 -> face illuminated/1
  If/1 -> If Action Subsystem/Action
  If Action Subsystem/1(Out1) -> Merge/1
  If/2 -> If Action Subsystem1/Action
  If Action Subsystem1/1(Out1) -> Merge/2
  If Action Subsystem4/1(Out1) -> Merge1/2
  If1/2 -> If Action Subsystem4/Action
  If1/1 -> If Action Subsystem3/Action
  If1/3 -> If Action Subsystem5/Action
  If Action Subsystem5/1(Out1) -> Merge1/3
  If Action Subsystem3/1(Out1) -> Merge1/1

== system Quaternions_Method_main_davide/Enviroment/Solar Radiation Perturbation/Torque_arm/creazione raggi vettore tra CM MB e centro facce illuminate della faccia che ha come normale l'asse i ==
  S_B : Inport
  MB : Inport  Port=2
  A_vect : Inport  Port=3
  pointer : Inport  Port=4
  Add2 : Sum  Inputs=+|+|+|+|+
  Demux1 : Demux  Outputs=3
  If Action Subsystem : Subsystem  TreatAsAtomicUnit=on
  If Action Subsystem1 : Subsystem  TreatAsAtomicUnit=on
  If Action Subsystem2 : Subsystem  TreatAsAtomicUnit=on
  If Action Subsystem3 : Subsystem  TreatAsAtomicUnit=on
  If Action Subsystem4 : Subsystem  TreatAsAtomicUnit=on
  If Action Subsystem5 : Subsystem  TreatAsAtomicUnit=on
  If Action Subsystem6 : Subsystem  TreatAsAtomicUnit=on
  If Action Subsystem8 : Subsystem  TreatAsAtomicUnit=on
  If1 : If  NumInputs=2  IfExpression=u1>0 & u2>0
  If2 : If  NumInputs=2  IfExpression=u1<0 & u2>0
  If3 : If  NumInputs=2  IfExpression=u1>0 & u2<0
  If4 : If  NumInputs=2  IfExpression=u1<0 & u2<0
  Merge{,1..3} (4 alike) : Merge
  Reshape1 : Reshape  OutputDimensionality=Column vector (2-D)
  Terminator1 : Terminator
  creating distance between cm MB and centro geom lato : Subsystem
  Out1 : Outport
  wires:
  [A_vect] -> If Action Subsystem2/1(Areas_vect)
  [A_vect] -> If Action Subsystem1/1(Areas_vect)
  [A_vect] -> If Action Subsystem4/1(Areas_vect)
  Add2/1 -> Out1/1
  Merge3/1 -> Add2/5  "raggio vettore centro geom lato- centro geom lato illuminato"
  If4/1 -> If Action Subsystem2/Action
  If Action Subsystem2/1(r_cface_cluce_yneg_z_neg) -> Merge3/1
  If3/1 -> If Action Subsystem1/Action
  [A_vect] -> If Action Subsystem/1(Areas_vect)
  Merge1/1 -> Add2/3  "raggio vettore centro geom lato- centro geom lato illuminato"
  If Action Subsystem4/1(r_cface_cluce_zneg_y_pos) -> Merge1/1
  Merge/1 -> Add2/2  "raggio vettore centro geom lato- centro geom lato illuminato"
  If Action Subsystem/1(r_cface_cluce_yz_pos) -> Merge/1
  If1/2 -> If Action Subsystem8/Action
  S_B/1 -> Reshape1/1
  Reshape1/1 -> Demux1/1
  Demux1/2 -> If2/2, If3/2, If4/2, If1/2  "S_B_y"
  If2/1 -> If Action Subsystem4/Action
  If1/1 -> If Action Subsystem/Action
  Demux1/3 -> If4/1, If3/1, If2/1, If1/1  "S_B_z"
  creating distance between cm MB and centro geom lato/1(Out1) -> Add2/1
  Demux1/1 -> Terminator1/1  "S_B_x"
  MB/1 -> [MB]
  [MB] -> If Action Subsystem/2(MB)
  [MB] -> If Action Subsystem4/2(MB)
  [MB] -> If Action Subsystem1/2(MB)
  [MB] -> If Action Subsystem2/2(MB)
  If Action Subsystem8/1(Out1) -> Merge/2
  If2/2 -> If Action Subsystem3/Action
  If3/2 -> If Action Subsystem5/Action
  If4/2 -> If Action Subsystem6/Action
  If Action Subsystem3/1(Out1) -> Merge1/2
  If Action Subsystem1/1(r_cface_cluce_yneg_z_pos) -> Merge2/1
  If Action Subsystem5/1(Out1) -> Merge2/2
  Merge2/1 -> Add2/4  "raggio vettore centro geom lato- centro geom lato illuminato"
  If Action Subsystem6/1(Out1) -> Merge3/2
  [MB] -> creating distance between cm MB and centro geom lato/1(MB)
  A_vect/1 -> [A_vect]
  pointer/1 -> creating distance between cm MB and centro geom lato/2(pointer)

== system Quaternions_Method_main_davide/Enviroment/Solar Radiation Perturbation/Torque_arm/creazione raggi vettore tra CM MB e centro facce illuminate della faccia che ha come normale l'asse j ==
  S_B : Inport
  MB : Inport  Port=2
  A_vect : Inport  Port=3
  pointer : Inport  Port=4
  Add2 : Sum  Inputs=+|+|+|+|+
  Demux1 : Demux  Outputs=3
  If Action Subsystem : Subsystem  TreatAsAtomicUnit=on
  If Action Subsystem1 : Subsystem  TreatAsAtomicUnit=on
  If Action Subsystem2 : Subsystem  TreatAsAtomicUnit=on
  If Action Subsystem3 : Subsystem  TreatAsAtomicUnit=on
  If Action Subsystem4 : Subsystem  TreatAsAtomicUnit=on
  If Action Subsystem5 : Subsystem  TreatAsAtomicUnit=on
  If Action Subsystem6 : Subsystem  TreatAsAtomicUnit=on
  If Action Subsystem7 : Subsystem  TreatAsAtomicUnit=on
  If1 : If  NumInputs=2  IfExpression=u1>0 & u2>0
  If2 : If  NumInputs=2  IfExpression=u1<0 & u2>0
  If3 : If  NumInputs=2  IfExpression=u1>0 & u2<0
  If4 : If  NumInputs=2  IfExpression=u1<0 & u2<0
  Merge{,1..3} (4 alike) : Merge
  Reshape1 : Reshape  OutputDimensionality=Column vector (2-D)
  Terminator1 : Terminator
  creating distance between cm MB and centro geom lato1 : Subsystem
  Out1 : Outport
  wires:
  Demux1/2 -> Terminator1/1
  creating distance between cm MB and centro geom lato1/1(Out1) -> Add2/1
  If1/1 -> If Action Subsystem/Action
  If2/1 -> If Action Subsystem1/Action
  Reshape1/1 -> Demux1/1
  S_B/1 -> Reshape1/1
  If Action Subsystem/1(r_cface_cluce_xz_pos) -> Merge/1
  Merge/1 -> Add2/2  "raggio vettore centro geom lato- centro geom lato illuminato"
  If Action Subsystem1/1(r_cface_cluce_x_pos_z_neg) -> Merge1/1
  Merge1/1 -> Add2/3  "raggio vettore centro geom lato- centro geom lato illuminato"
  [A_vect] -> If Action Subsystem/1(Areas_vect)
  Merge2/1 -> Add2/4  "raggio vettore centro geom lato- centro geom lato illuminato"
  If3/1 -> If Action Subsystem2/Action
  If Action Subsystem3/1(r_cface_cluce_x_neg_z_neg) -> Merge3/1
  If4/1 -> If Action Subsystem3/Action
  Merge3/1 -> Add2/5  "raggio vettore centro geom lato- centro geom lato illuminato"
  Add2/1 -> Out1/1
  [A_vect] -> If Action Subsystem1/1(Areas_vect)
  [A_vect] -> If Action Subsystem2/1(Areas_vect)
  [A_vect] -> If Action Subsystem3/1(Areas_vect)
  Demux1/3 -> If4/1, If3/1, If2/1, If1/1  "S_B_z"
  Demux1/1 -> If1/2, If4/2, If3/2, If2/2  "S_B_x"
  MB/1 -> [MB]
  [MB] -> If Action Subsystem/2(MB)
  [MB] -> If Action Subsystem1/2(MB)
  [MB] -> If Action Subsystem2/2(MB)
  [MB] -> If Action Subsystem3/2(MB)
  If1/2 -> If Action Subsystem5/Action
  If2/2 -> If Action Subsystem4/Action
  If3/2 -> If Action Subsystem6/Action
  If4/2 -> If Action Subsystem7/Action
  If Action Subsystem5/1(Out1) -> Merge/2
  If Action Subsystem4/1(Out1) -> Merge1/2
  If Action Subsystem2/1(r_cface_cluce_x_neg_z_pos) -> Merge2/1
  If Action Subsystem6/1(Out1) -> Merge2/2
  If Action Subsystem7/1(Out1) -> Merge3/2
  [MB] -> creating distance between cm MB and centro geom lato1/1(MB)
  A_vect/1 -> [A_vect]
  pointer/1 -> creating distance between cm MB and centro geom lato1/2(pointer)

== system Quaternions_Method_main_davide/Enviroment/Solar Radiation Perturbation/Torque_arm/creazione raggi vettore tra CM MB e centro facce illuminate della faccia che ha come normale l'asse k ==
  S_B : Inport
  MB : Inport  Port=2
  A_vect : Inport  Port=3
  pointer : Inport  Port=4
  Add2 : Sum  Inputs=+|+|+|+|+
  Demux1 : Demux  Outputs=3
  If Action Subsystem : Subsystem  TreatAsAtomicUnit=on
  If Action Subsystem1 : Subsystem  TreatAsAtomicUnit=on
  If Action Subsystem2 : Subsystem  TreatAsAtomicUnit=on
  If Action Subsystem3 : Subsystem  TreatAsAtomicUnit=on
  If Action Subsystem4 : Subsystem  TreatAsAtomicUnit=on
  If Action Subsystem5 : Subsystem  TreatAsAtomicUnit=on
  If Action Subsystem6 : Subsystem  TreatAsAtomicUnit=on
  If Action Subsystem7 : Subsystem  TreatAsAtomicUnit=on
  If1 : If  NumInputs=2  IfExpression=u1>0 & u2>0
  If2 : If  NumInputs=2  IfExpression=u1<0 & u2>0
  If3 : If  NumInputs=2  IfExpression=u1>0 & u2<0
  If4 : If  NumInputs=2  IfExpression=u1<0 & u2<0
  Merge{,1..3} (4 alike) : Merge
  Reshape1 : Reshape  OutputDimensionality=Column vector (2-D)
  Terminator1 : Terminator
  creating distance between cm MB and centro geom lato1 : Subsystem
  Out1 : Outport
  wires:
  Demux1/3 -> Terminator1/1
  Demux1/1 -> If1/1, If4/1, If3/1, If2/1  "S_B_x"
  If1/1 -> If Action Subsystem/Action
  If2/1 -> If Action Subsystem4/Action
  Demux1/2 -> If4/2, If3/2, If2/2, If1/2  "S_B_y"
  Reshape1/1 -> Demux1/1
  S_B/1 -> Reshape1/1
  If1/2 -> If Action Subsystem5/Action
  Merge/1 -> Add2/2  "raggio vettore centro geom lato- centro geom lato illuminato"
  Merge1/1 -> Add2/3  "raggio vettore centro geom lato- centro geom lato illuminato"
  [A_vect] -> If Action Subsystem/1(Areas_vect)
  Merge2/1 -> Add2/4  "raggio vettore centro geom lato- centro geom lato illuminato"
  If3/2 -> If Action Subsystem6/Action
  If Action Subsystem1/1(r_cface_cluce_xpos_y_neg) -> Merge2/1
  If3/1 -> If Action Subsystem1/Action
  If4/2 -> If Action Subsystem7/Action
  If4/1 -> If Action Subsystem2/Action
  Merge3/1 -> Add2/5  "raggio vettore centro geom lato- centro geom lato illuminato"
  Add2/1 -> Out1/1
  [A_vect] -> If Action Subsystem4/1(Areas_vect)
  [A_vect] -> If Action Subsystem1/1(Areas_vect)
  [A_vect] -> If Action Subsystem2/1(Areas_vect)
  MB/1 -> [MB]
  [MB] -> If Action Subsystem/2(MB)
  [MB] -> If Action Subsystem4/2(MB1)
  [MB] -> If Action Subsystem1/2(MB)
  [MB] -> If Action Subsystem2/2(MB1)
  If2/2 -> If Action Subsystem3/Action
  If Action Subsystem/1(r_cface_cluce_xy_pos) -> Merge/1
  If Action Subsystem5/1(Out1) -> Merge/2
  If Action Subsystem4/1(r_cface_cluce_xneg_y_pos) -> Merge1/1
  If Action Subsystem3/1(Out1) -> Merge1/2
  If Action Subsystem6/1(Out1) -> Merge2/2
  If Action Subsystem2/1(r_cface_cluce_xneg_y_neg) -> Merge3/1
  If Action Subsystem7/1(Out1) -> Merge3/2
  [MB] -> creating distance between cm MB and centro geom lato1/1(MB)
  creating distance between cm MB and centro geom lato1/1(Out1) -> Add2/1
  A_vect/1 -> [A_vect]
  pointer/1 -> creating distance between cm MB and centro geom lato1/2(pointer)

== system Quaternions_Method_main_davide/Kinematics1/Creazione quaternione/DCM to quaternion/Case 1 ==
  A11 : Inport
  A22 : Inport  Port=2
  A33 : Inport  Port=3
  Add : Sum  Inputs=++--
  Constant : Constant
  Gain : Gain  Gain=1/2
  Sqrt : Sqrt  SaturateOnIntegerOverflow=on
  q1 : Outport
  wires:
  A22/1 -> Add/3
  A11/1 -> Add/2
  A33/1 -> Add/4
  Constant/1 -> Add/1
  Add/1 -> Sqrt/1
  Sqrt/1 -> Gain/1
  Gain/1 -> q1/1

== system Quaternions_Method_main_davide/Kinematics1/Creazione quaternione/DCM to quaternion/Case 2 ==
  A11 : Inport
  A22 : Inport  Port=2
  A33 : Inport  Port=3
  Add : Sum  Inputs=+-+-
  Constant : Constant
  Gain : Gain  Gain=1/2
  Sqrt : Sqrt  SaturateOnIntegerOverflow=on
  q2 : Outport
  wires:
  Gain/1 -> q2/1
  Sqrt/1 -> Gain/1
  Add/1 -> Sqrt/1
  Constant/1 -> Add/1
  A33/1 -> Add/4
  A11/1 -> Add/2
  A22/1 -> Add/3

== system Quaternions_Method_main_davide/Kinematics1/Creazione quaternione/DCM to quaternion/Case 3 ==
  A11 : Inport
  A22 : Inport  Port=2
  A33 : Inport  Port=3
  Add : Sum  Inputs=+--+
  Constant : Constant
  Gain : Gain  Gain=1/2
  Sqrt : Sqrt  SaturateOnIntegerOverflow=on
  q3 : Outport
  wires:
  A22/1 -> Add/3
  A11/1 -> Add/2
  A33/1 -> Add/4
  Constant/1 -> Add/1
  Add/1 -> Sqrt/1
  Sqrt/1 -> Gain/1
  Gain/1 -> q3/1

== system Quaternions_Method_main_davide/Kinematics1/Creazione quaternione/DCM to quaternion/Case 4 ==
  A11 : Inport
  A22 : Inport  Port=2
  A33 : Inport  Port=3
  Add : Sum  Inputs=++++
  Constant : Constant
  Gain : Gain  Gain=1/2
  Sqrt : Sqrt  SaturateOnIntegerOverflow=on
  q4 : Outport
  wires:
  Gain/1 -> q4/1
  Sqrt/1 -> Gain/1
  Add/1 -> Sqrt/1
  Constant/1 -> Add/1
  A33/1 -> Add/4
  A11/1 -> Add/2
  A22/1 -> Add/3

== system Quaternions_Method_main_davide/Kinematics1/Creazione quaternione/DCM to quaternion/If Action Subsystem ==
  In2 : Inport
  In1 : Inport  Port=2
  Action Port : ActionPort
  Add : Sum
  Add1 : Sum
  Add2 : Sum  Inputs=+-
  Demux : Demux  Outputs=6
  Gain : Gain  Gain=4
  Mux : Mux
  Product : Product
  Product1 : Product
  Product2 : Product
  Reciprocal : Product  Inputs=/
  Reshape : Reshape  OutputDimensionality=Column vector (2-D)
  q_vect1 : Outport
  wires:
  In1/1 -> Demux/1
  In2/1 -> [q1]
  Mux/1 -> Reshape/1
  Reshape/1 -> q_vect1/1
  [q1] -> Mux/1
  Demux/3 -> [A12]
  Demux/2 -> [A31]
  Demux/1 -> [A21]
  Demux/6 -> [A23]
  Demux/5 -> [A13]
  Demux/4 -> [A32]
  [q1] -> Gain/1
  Gain/1 -> Reciprocal/1
  Reciprocal/1 -> [q1_div]
  Add/1 -> Product/1
  [A21] -> Add/2
  [A12] -> Add/1
  [q1_div] -> Product/2
  Product/1 -> [q2]
  Product1/1 -> [q3]
  [q1_div] -> Product1/2
  [A13] -> Add1/1
  [A31] -> Add1/2
  Add1/1 -> Product1/1
  Add2/1 -> Product2/1
  [A32] -> Add2/2
  [A23] -> Add2/1
  [q1_div] -> Product2/2
  Product2/1 -> [q4]
  [q2] -> Mux/2
  [q3] -> Mux/3
  [q4] -> Mux/4

== system Quaternions_Method_main_davide/Kinematics1/Creazione quaternione/DCM to quaternion/If Action Subsystem1 ==
  In2 : Inport
  In1 : Inport  Port=2
  Action Port : ActionPort
  Add : Sum
  Add1 : Sum  Inputs=-+
  Add2 : Sum
  Demux : Demux  Outputs=6
  Gain : Gain  Gain=4
  Mux : Mux
  Product : Product
  Product1 : Product
  Product2 : Product
  Reciprocal : Product  Inputs=/
  Reshape : Reshape  OutputDimensionality=Column vector (2-D)
  q_vect2 : Outport
  wires:
  [q4] -> Mux/4
  [q3] -> Mux/3
  [q2] -> Mux/2
  Product2/1 -> [q3]
  [q2_div] -> Product2/2
  [A23] -> Add2/1
  [A32] -> Add2/2
  Add2/1 -> Product2/1
  Add1/1 -> Product1/1
  [A31] -> Add1/2
  [A13] -> Add1/1
  [q2_div] -> Product1/2
  Product1/1 -> [q4]
  Product/1 -> [q1]
  [q2_div] -> Product/2
  [A12] -> Add/1
  [A21] -> Add/2
  Add/1 -> Product/1
  Reciprocal/1 -> [q2_div]
  Gain/1 -> Reciprocal/1
  [q2] -> Gain/1
  Demux/4 -> [A32]
  Demux/5 -> [A13]
  Demux/6 -> [A23]
  Demux/1 -> [A21]
  Demux/2 -> [A31]
  Demux/3 -> [A12]
  [q1] -> Mux/1
  Reshape/1 -> q_vect2/1
  Mux/1 -> Reshape/1
  In2/1 -> [q2]
  In1/1 -> Demux/1

== system Quaternions_Method_main_davide/Kinematics1/Creazione quaternione/DCM to quaternion/If Action Subsystem2 ==
  In2 : Inport
  In1 : Inport  Port=2
  Action Port : ActionPort
  Add : Sum  Inputs=+-
  Add1 : Sum
  Add2 : Sum  Inputs=+-
  Demux : Demux  Outputs=6
  Gain : Gain  Gain=4
  Mux : Mux
  Product : Product
  Product1 : Product
  Product2 : Product
  Reciprocal : Product  Inputs=/
  Reshape : Reshape  OutputDimensionality=Column vector (2-D)
  q_vect3 : Outport
  wires:
  In1/1 -> Demux/1
  In2/1 -> [q3]
  Mux/1 -> Reshape/1
  Reshape/1 -> q_vect3/1
  [q1] -> Mux/1
  Demux/3 -> [A12]
  Demux/2 -> [A31]
  Demux/1 -> [A21]
  Demux/6 -> [A23]
  Demux/5 -> [A13]
  Demux/4 -> [A32]
  [q3] -> Gain/1
  Gain/1 -> Reciprocal/1
  Reciprocal/1 -> [q3_div]
  Add/1 -> Product/1
  [A21] -> Add/2
  [A12] -> Add/1
  [q3_div] -> Product/2
  Product/1 -> [q4]
  Product1/1 -> [q1]
  [q3_div] -> Product1/2
  [A13] -> Add1/1
  [A31] -> Add1/2
  Add1/1 -> Product1/1
  Add2/1 -> Product2/1
  [A32] -> Add2/2
  [A23] -> Add2/1
  [q3_div] -> Product2/2
  Product2/1 -> [q2]
  [q2] -> Mux/2
  [q3] -> Mux/3
  [q4] -> Mux/4

== system Quaternions_Method_main_davide/Kinematics1/Creazione quaternione/DCM to quaternion/If Action Subsystem3 ==
  In2 : Inport
  In1 : Inport  Port=2
  Action Port : ActionPort
  Add : Sum  Inputs=+-
  Add1 : Sum  Inputs=-+
  Add2 : Sum  Inputs=+-
  Demux : Demux  Outputs=6
  Gain : Gain  Gain=4
  Mux : Mux
  Product : Product
  Product1 : Product
  Product2 : Product
  Reciprocal : Product  Inputs=/
  Reshape : Reshape  OutputDimensionality=Column vector (2-D)
  q_vect4 : Outport
  wires:
  [q4] -> Mux/4
  [q3] -> Mux/3
  [q2] -> Mux/2
  Product2/1 -> [q1]
  [q4_div] -> Product2/2
  [A23] -> Add2/1
  [A32] -> Add2/2
  Add2/1 -> Product2/1
  Add1/1 -> Product1/1
  [A31] -> Add1/2
  [A13] -> Add1/1
  [q4_div] -> Product1/2
  Product1/1 -> [q2]
  Product/1 -> [q3]
  [q4_div] -> Product/2
  [A12] -> Add/1
  [A21] -> Add/2
  Add/1 -> Product/1
  Reciprocal/1 -> [q4_div]
  Gain/1 -> Reciprocal/1
  [q4] -> Gain/1
  Demux/4 -> [A32]
  Demux/5 -> [A13]
  Demux/6 -> [A23]
  Demux/1 -> [A21]
  Demux/2 -> [A31]
  Demux/3 -> [A12]
  [q1] -> Mux/1
  Reshape/1 -> q_vect4/1
  Mux/1 -> Reshape/1
  In2/1 -> [q4]
  In1/1 -> Demux/1

== system Quaternions_Method_main_davide/Kinematics1/Relative_Attitude/A_LN/M1 ==
  Input : Inport
  Constant{1..2,4..5} (4 alike) : Constant  Value=0
  Constant3 : Constant
  Cos : Trigonometry  Operator=cos
  Cos1 : Trigonometry
  Cos2 : Trigonometry  Operator=cos
  Cos3 : Trigonometry
  Matrix Concatenate : Concatenate  NumInputs=3  Mode=Multidimensional array  ConcatenateDimension=2
  Multiply : Gain  Gain=-1
  Mux : Mux  Inputs=3
  Mux1 : Mux  Inputs=3
  Mux2 : Mux  Inputs=3
  Reshape : Reshape  OutputDimensionality=Column vector (2-D)
  Reshape1 : Reshape  OutputDimensionality=Column vector (2-D)
  Reshape2 : Reshape  OutputDimensionality=Column vector (2-D)
  Out1 : Outport
  wires:
  Multiply/1 -> Mux/2
  Cos/1 -> Mux/1
  Constant1/1 -> Mux/3
  Constant2/1 -> Mux1/3
  Input/1 -> Cos/1, Cos1/1, Cos3/1, Cos2/1
  Matrix Concatenate/1 -> Out1/1
  Cos3/1 -> Mux1/1
  Constant5/1 -> Mux2/1
  Cos2/1 -> Mux1/2
  Constant3/1 -> Mux2/3
  Constant4/1 -> Mux2/2
  Cos1/1 -> Multiply/1
  Mux/1 -> Reshape/1
  Reshape/1 -> Matrix Concatenate/1
  Reshape1/1 -> Matrix Concatenate/2
  Mux1/1 -> Reshape1/1
  Mux2/1 -> Reshape2/1
  Reshape2/1 -> Matrix Concatenate/3

== system Quaternions_Method_main_davide/Kinematics1/Relative_Attitude/A_LN/M2 ==
  ii : Inport
  Constant{1..4} (4 alike) : Constant  Value=0
  Constant5 : Constant
  Cos : Trigonometry  Operator=cos
  Cos1 : Trigonometry
  Cos2 : Trigonometry  Operator=cos
  Cos3 : Trigonometry
  Matrix Concatenate : Concatenate  NumInputs=3  Mode=Multidimensional array  ConcatenateDimension=2
  Multiply : Gain  Gain=-1
  Mux : Mux  Inputs=3
  Mux1 : Mux  Inputs=3
  Mux2 : Mux  Inputs=3
  Reshape : Reshape  OutputDimensionality=Column vector (2-D)
  Reshape1 : Reshape  OutputDimensionality=Column vector (2-D)
  Reshape2 : Reshape  OutputDimensionality=Column vector (2-D)
  Out1 : Outport
  wires:
  Matrix Concatenate/1 -> Out1/1
  Constant5/1 -> Mux2/1
  Constant3/1 -> Mux2/3
  Constant4/1 -> Mux2/2
  Cos1/1 -> Multiply/1
  Constant1/1 -> Mux/1
  Cos/1 -> Mux/2
  Multiply/1 -> Mux/3
  Constant2/1 -> Mux1/1
  Cos3/1 -> Mux1/2
  Cos2/1 -> Mux1/3
  ii/1 -> Cos2/1, Cos/1, Cos1/1, Cos3/1
  Mux2/1 -> Reshape/1
  Reshape/1 -> Matrix Concatenate/1
  Mux/1 -> Reshape1/1
  Reshape1/1 -> Matrix Concatenate/2
  Reshape2/1 -> Matrix Concatenate/3
  Mux1/1 -> Reshape2/1
